simulink model "Arm6Dof"  (R2018b)
settings: Solver=VariableStepAuto  StartTime=0.0  StopTime=inf  RelTol=1e-3
undefined symbols (not defined in the file or in its folder): asm_Arm6Dof, bottom, link1, link2, link3, link4, link5, linke, RootGround, RootPart
libraries: mblibv1 x25, simulink x7
settings Model: Creator=Administrator  LastModifiedBy=Administrator
settings SimMechanicsCC: VisOnUpdateDiagram=on  VisDuringSimulation=on

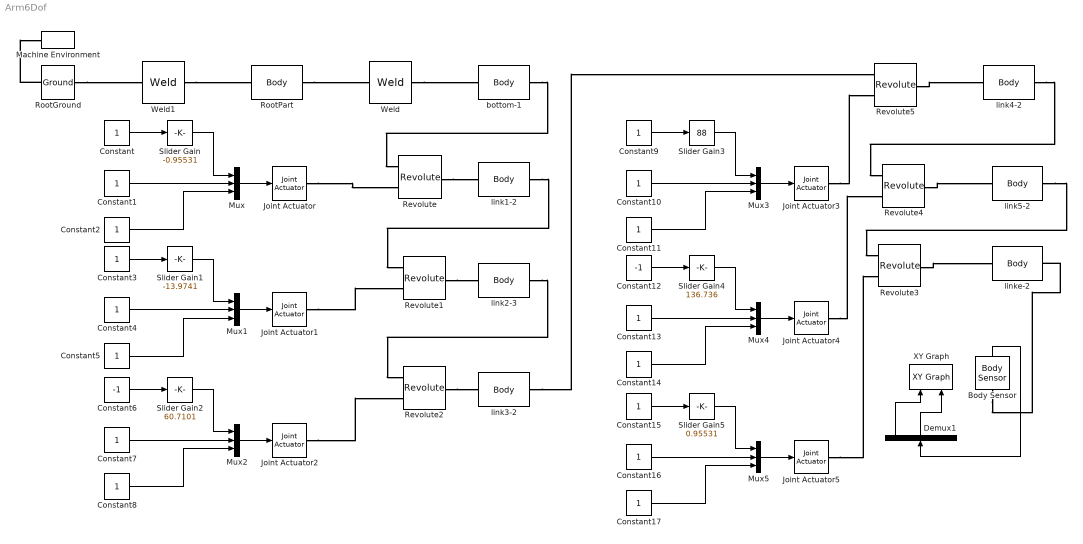
== system Arm6Dof ==
  Body Sensor : mblibv1/Sensors &  Actuators/Body Sensor  UpdateFromCAD=off  PhysicalDomain=Mechanical  PortType=blob  Muxed=on  Pose=off  Angle=on  AngleUnits=deg  ArcVelocity=off  ArcVelocityUnits=deg/s  ArcAcceleration=off  ArcAccelerationUnits=deg/s^2  CoordPosition=on  CoordPositionUnits=mm  Velocity=off  VelocityUnits=m/s  Acceleration=off  AccelerationUnits=m/s^2  Quaternion=on  QuaternionDT=off  QuaternionDDT=off  QuaternionUnits=off  OutputVector=[1]  ActiveIO=on  Width=3  DialogClass=MechanicalSensorBlock  ReferenceFrame=Absolute (World)
      settings: SourceProductName=Simscape  SourceProductBaseCode=SS
  Constant{,1..5,7..11,13..17} (16 alike) : Constant
  Constant12 : Constant  Value=-1
  Constant6 : Constant  Value=-1
  Demux1 : Demux  Outputs=3
  Joint Actuator{,1..5} (6 alike) : mblibv1/Sensors &  Actuators/Joint Actuator  UpdateFromCAD=off  PhysicalDomain=Mechanical  PortType=blob  ActuationStyle=Motion  AngleUnits=deg  ArcVelocityUnits=deg/s  ArcAccelerationUnits=deg/s^2  CoordPositionUnits=m  VelocityUnits=m/s  AccelerationUnits=m/s^2  ForceUnits=N  TorqueUnits=N*m  ActiveIO=on  Width=3  DialogClass=MechanicalActuatorBlock  Primitive=R1  ReferenceFrame=Absolute (World)
      settings: SourceProductName=Simscape  SourceProductBaseCode=SS
  Machine Environment : mblibv1/Bodies/Machine Environment  PortType=env  PhysicalDomain=Mechanical  DialogTemplateClass=MECH.MachineEnvironment  SyncWhenCopied=off  Gravity=[0 -9.81 0]  GravityUnits=m/s^2  GravityAsSignal=off  Dimensionality=Auto-detect  AnalysisType=Forward dynamics  LinearAssemblyTolerance=1e-3  LinearAssemblyToleranceUnits=m  AngularAssemblyTolerance=1e-3  AngularAssemblyToleranceUnits=rad  ConstraintSolverType=Stabilizing  ConstraintRelTolerance=1e-4  ConstraintAbsTolerance=1e-4  UseRobustSingularityHandling=off  RedundancyAnalysisToleranceType=Automatically select tolerance  RedundancyAnalysisTolerance=1e-14  StatePerturbationType=Fixed  PerturbationSize=1e-5  VisualizeMachine=on  BodyVisualizationType=Use model default body geometries  BodyColorSelMode=Use model default  DefaultBodyColor=[1 0 0]
      settings: SourceProductName=Simscape  SourceProductBaseCode=SS
  Mux{,1..5} (6 alike) : Mux  Inputs=3
  Revolute : mblibv1/Joints/Revolute  LConnTagsString=__newl0|SA1  RConnTagsString=__newr0  UpdateFromCAD=on  PMImportedID=bottom-1:-:link1-2  NumSAPorts=1  CutJoint=off  MarkAsCut=off  Primitives=prismatic  PrimitiveProps=R1$World$[0,0,1]$revolute  DialogClass=JointBlock  R1Axis=[0,0,1]
      settings: SourceProductName=Simscape  SourceProductBaseCode=SS
  Revolute1 : mblibv1/Joints/Revolute  LConnTagsString=__newl0|SA1  RConnTagsString=__newr0  UpdateFromCAD=on  PMImportedID=link1-2:-:link2-3  NumSAPorts=1  CutJoint=off  MarkAsCut=off  Primitives=prismatic  PrimitiveProps=R1$World$[0,1,0]$revolute  DialogClass=JointBlock  R1Axis=[0,1,0]
      settings: SourceProductName=Simscape  SourceProductBaseCode=SS
  Revolute2 : mblibv1/Joints/Revolute  LConnTagsString=__newl0|SA1  RConnTagsString=__newr0  UpdateFromCAD=on  PMImportedID=link2-3:-:link3-2  NumSAPorts=1  CutJoint=off  MarkAsCut=off  Primitives=prismatic  PrimitiveProps=R1$World$[0,-1,0]$revolute  DialogClass=JointBlock  R1Axis=[0,-1,0]
      settings: SourceProductName=Simscape  SourceProductBaseCode=SS
  Revolute3 : mblibv1/Joints/Revolute  LConnTagsString=__newl0|SA1  RConnTagsString=__newr0  UpdateFromCAD=on  PMImportedID=link5-2:-:linke-2  NumSAPorts=1  CutJoint=off  MarkAsCut=off  Primitives=prismatic  PrimitiveProps=R1$World$[1,0,0]$revolute  DialogClass=JointBlock  R1Axis=[1,0,0]
      settings: SourceProductName=Simscape  SourceProductBaseCode=SS
  Revolute4 : mblibv1/Joints/Revolute  LConnTagsString=__newl0|SA1  RConnTagsString=__newr0  UpdateFromCAD=on  PMImportedID=link4-2:-:link5-2  NumSAPorts=1  CutJoint=off  MarkAsCut=off  Primitives=prismatic  PrimitiveProps=R1$World$[0,-1,0]$revolute  DialogClass=JointBlock  R1Axis=[0,-1,0]
      settings: SourceProductName=Simscape  SourceProductBaseCode=SS
  Revolute5 : mblibv1/Joints/Revolute  LConnTagsString=__newl0|SA1  RConnTagsString=__newr0  UpdateFromCAD=on  PMImportedID=link3-2:-:link4-2  NumSAPorts=1  CutJoint=off  MarkAsCut=off  Primitives=prismatic  PrimitiveProps=R1$World$[1,0,0]$revolute  DialogClass=JointBlock  R1Axis=[1,0,0]
      settings: SourceProductName=Simscape  SourceProductBaseCode=SS
  RootGround : mblibv1/Bodies/Ground  UpdateFromCAD=on  PMImportedID=RootGround  LeftPortType=env  RightPortType=workingframe  PhysicalDomain=Mechanical  DialogClass=GroundBlock  CoordPosition=[0.0237894,0.00138772,0.108536]  CoordPositionUnits=m  StateVectorMgrId=0  MachineId=[1 0]  ShowEnvPort=on  ParameterChecksum=[465685806, 464748915, 4149600887, 3518869036]  TopologyChecksum=[603143340, 271073404, 1386402031, 4009897821]
      settings: SourceProductName=Simscape  SourceProductBaseCode=SS
  RootPart : mblibv1/Bodies/Body  LConnTagsString=CS3  RConnTagsString=CS2  UpdateFromCAD=on  PMImportedID=asm_Arm6Dof/RootPart  DialogClass=MechanicalBodyBlock  Mass=0  MassUnits=kg  InertiaUnits=kg*m^2  Inertia=[0,0,0;0,0,0;0,0,0]  Shape=Cylinder  ShapeDims=[1 1]  ShapeUnits=m  ShapeUse=false  Density=1  DensityUnits=kg/m^3  DensityUse=false  GraphicsMode=MACHINE_DEFAULT  BodyColorSelMode=MACHINE_DEFAULT  BodyColor=[1;0;0]  AttachedToCS=CS1  CG=Right$CG$[0.0237894 0.00138772 0.108536]$WORLD$WORLD$m$[1 0 0;0 1 0;0 0 1]$3x3 Transform$rad$WORLD$false$asm_Arm6Dof/RootPart::CG(AUTOGEN)  WorkingFrames=Right$CS1$[0 0 0]$WORLD$WORLD$m$[1 0 0;0 1 0;0 0 1]$3x3 Transform$rad$WORLD$false$asm_Arm6Dof/RootPart::CS1(AUTOGEN)#Right$CS2$[0 0 0.005]$WORLD$WORLD$m$[1 0 0;0 1 0;0 0 1]$3x3 Transform$rad$WORLD$true$asm_Arm6Dof/RootPart:-:bottom-1::asm_Arm6Dof/RootPart(AUTOGEN)#Left$CS3$[0.0237894 0.00138772 0.108536]$WORLD$WORLD$m$[1 0 0;0 1 0;0 0 1]$3x3 Transform$rad$WORLD$true$RootGround:-:asm_Arm6Dof/RootPart::asm_Arm6Dof/RootPart(AUTOGEN)  CGPos=[0.0237894 0.00138772 0.108536]  CGRot=[1 0 0;0 1 0;0 0 1]  CS0Pos=[]  CS0Rot=[]  CS1Pos=[0 0 0]  CS1Rot=[1 0 0;0 1 0;0 0 1]  CS2Pos=[0 0 0.005]  CS2Rot=[1 0 0;0 1 0;0 0 1]  CS3Pos=[0.0237894 0.00138772 0.108536]  CS3Rot=[1 0 0;0 1 0;0 0 1]  CS4Pos=[]  CS4Rot=[]  CS5Pos=[]  CS5Rot=[]  CS6Pos=[]  CS6Rot=[]  CS7Pos=[]  CS7Rot=[]  CS8Pos=[]  CS8Rot=[]  CS9Pos=[]  CS9Rot=[]  CS10Pos=[]  CS10Rot=[]  CS11Pos=[]  CS11Rot=[]  CS12Pos=[]  CS12Rot=[]  CS13Pos=[]  CS13Rot=[]  CS14Pos=[]  CS14Rot=[]  CS15Pos=[]  CS15Rot=[]  CS16Pos=[]  CS16Rot=[]  CS17Pos=[]  CS17Rot=[]  CS18Pos=[]  CS18Rot=[]  CS19Pos=[]  CS19Rot=[]  CS20Pos=[]  CS20Rot=[]
      settings: SourceProductName=Simscape  SourceProductBaseCode=SS
  Slider Gain : simulink/Math Operations/Slider Gain  gain=-0.95531  low=-180  high=180
  Slider Gain1 : simulink/Math Operations/Slider Gain  gain=-13.9741  low=-180  high=180
  Slider Gain2 : simulink/Math Operations/Slider Gain  gain=60.7101  low=-180  high=180
  Slider Gain3 : simulink/Math Operations/Slider Gain  gain=88  low=-180  high=180
  Slider Gain4 : simulink/Math Operations/Slider Gain  gain=136.736  low=-180  high=180
  Slider Gain5 : simulink/Math Operations/Slider Gain  gain=0.95531  low=-180  high=180
  Weld : mblibv1/Joints/Weld  LConnTagsString=__newl0  RConnTagsString=__newr0  UpdateFromCAD=on  PMImportedID=asm_Arm6Dof/RootPart:-:bottom-1  NumSAPorts=0  CutJoint=off  MarkAsCut=off  Primitives=weld  PrimitiveProps=W$WORLD$[0.57735,0.57735,0.57735]$weld  DialogClass=JointBlock  WAxis=[0.57735,0.57735,0.57735]
      settings: SourceProductName=Simscape  SourceProductBaseCode=SS
  Weld1 : mblibv1/Joints/Weld  LConnTagsString=__newl0  RConnTagsString=__newr0  UpdateFromCAD=on  PMImportedID=RootGround:-:asm_Arm6Dof/RootPart  NumSAPorts=0  CutJoint=off  MarkAsCut=off  Primitives=weld  PrimitiveProps=W$WORLD$[0.57735,0.57735,0.57735]$weld  DialogClass=JointBlock  WAxis=[0.57735,0.57735,0.57735]
      settings: SourceProductName=Simscape  SourceProductBaseCode=SS
  XY Graph : simulink/Sinks/XY Graph  xmin=-300  xmax=300  ymin=-300  ymax=300  st=1
  bottom-1 : mblibv1/Bodies/Body  LConnTagsString=CS2  RConnTagsString=CS3  UpdateFromCAD=on  PMImportedID=bottom-1  DialogClass=MechanicalBodyBlock  Mass=0.0989551  MassUnits=kg  InertiaUnits=kg*m^2  Inertia=[8.41493e-05,0,0;0,8.41493e-05,0;0,0,0.000166649]  Shape=Cylinder  ShapeDims=[1 1]  ShapeUnits=m  ShapeUse=false  Density=1  DensityUnits=kg/m^3  DensityUse=false  GraphicsMode=GFXFILE  GraphicsFileName=asm_Arm6Dof - bottom-1.STL  BodyColorSelMode=COLORPALETTE  BodyColor=[0.752941;0.752941;0.752941]  AttachedToCS=CS1  CG=Right$CG$[0 0 0.005]$WORLD$WORLD$m$[1 0 0;0 1 0;0 0 1]$3x3 Transform$rad$WORLD$false$bottom-1::CG(AUTOGEN)  WorkingFrames=Right$CS1$[0 0 0]$WORLD$WORLD$m$[1 0 0;0 1 0;0 0 1]$3x3 Transform$rad$WORLD$false$bottom-1::CS1(AUTOGEN)#Left$CS2$[0 0 0.005]$WORLD$WORLD$m$[1 0 0;0 1 0;0 0 1]$3x3 Transform$rad$WORLD$true$asm_Arm6Dof/RootPart:-:bottom-1::bottom-1(AUTOGEN)#Right$CS3$[0 0 0.01]$WORLD$WORLD$m$[1 0 0;0 1 0;0 0 1]$3x3 Transform$rad$WORLD$true$bottom-1:-:link1-2::bottom-1(AUTOGEN)  CGPos=[0 0 0.005]  CGRot=[1 0 0;0 1 0;0 0 1]  CS0Pos=[]  CS0Rot=[]  CS1Pos=[0 0 0]  CS1Rot=[1 0 0;0 1 0;0 0 1]  CS2Pos=[0 0 0.005]  CS2Rot=[1 0 0;0 1 0;0 0 1]  CS3Pos=[0 0 0.01]  CS3Rot=[1 0 0;0 1 0;0 0 1]  CS4Pos=[]  CS4Rot=[]  CS5Pos=[]  CS5Rot=[]  CS6Pos=[]  CS6Rot=[]  CS7Pos=[]  CS7Rot=[]  CS8Pos=[]  CS8Rot=[]  CS9Pos=[]  CS9Rot=[]  CS10Pos=[]  CS10Rot=[]  CS11Pos=[]  CS11Rot=[]  CS12Pos=[]  CS12Rot=[]  CS13Pos=[]  CS13Rot=[]  CS14Pos=[]  CS14Rot=[]  CS15Pos=[]  CS15Rot=[]  CS16Pos=[]  CS16Rot=[]  CS17Pos=[]  CS17Rot=[]  CS18Pos=[]  CS18Rot=[]  CS19Pos=[]  CS19Rot=[]  CS20Pos=[]  CS20Rot=[]
      settings: SourceProductName=Simscape  SourceProductBaseCode=SS
  link1-2 : mblibv1/Bodies/Body  LConnTagsString=CS2  RConnTagsString=CS3  UpdateFromCAD=on  PMImportedID=link1-2  DialogClass=MechanicalBodyBlock  Mass=0.27764  MassUnits=kg  InertiaUnits=kg*m^2  Inertia=[0.000579936,9.11984e-05,0;9.11984e-05,0.000159357,0;0,0,0.000651379]  Shape=Cylinder  ShapeDims=[1 1]  ShapeUnits=m  ShapeUse=false  Density=1  DensityUnits=kg/m^3  DensityUse=false  GraphicsMode=GFXFILE  GraphicsFileName=asm_Arm6Dof - link1-2.STL  BodyColorSelMode=COLORPALETTE  BodyColor=[1;0.152941;0.027451]  AttachedToCS=CS1  CG=Right$CG$[0.00665144 0 0.0836156]$WORLD$WORLD$m$[1 0 0;0 0 1;0 -1 0]$3x3 Transform$rad$WORLD$false$link1-2::CG(AUTOGEN)  WorkingFrames=Right$CS1$[0.047 0 0.133]$WORLD$WORLD$m$[1 0 0;0 0 1;0 -1 0]$3x3 Transform$rad$WORLD$false$link1-2::CS1(AUTOGEN)#Left$CS2$[0 0 0.01]$WORLD$WORLD$m$[1 0 0;0 1 0;0 0 1]$3x3 Transform$rad$WORLD$true$bottom-1:-:link1-2::link1-2(AUTOGEN)#Right$CS3$[0.047 -0.0055 0.133]$WORLD$WORLD$m$[1 0 0;0 1 0;0 0 1]$3x3 Transform$rad$WORLD$true$link1-2:-:link2-3::link1-2(AUTOGEN)  CGPos=[0.00665144 0 0.0836156]  CGRot=[1 0 0;0 0 1;0 -1 0]  CS0Pos=[]  CS0Rot=[]  CS1Pos=[0.047 0 0.133]  CS1Rot=[1 0 0;0 0 1;0 -1 0]  CS2Pos=[0 0 0.01]  CS2Rot=[1 0 0;0 1 0;0 0 1]  CS3Pos=[0.047 -0.0055 0.133]  CS3Rot=[1 0 0;0 1 0;0 0 1]  CS4Pos=[]  CS4Rot=[]  CS5Pos=[]  CS5Rot=[]  CS6Pos=[]  CS6Rot=[]  CS7Pos=[]  CS7Rot=[]  CS8Pos=[]  CS8Rot=[]  CS9Pos=[]  CS9Rot=[]  CS10Pos=[]  CS10Rot=[]  CS11Pos=[]  CS11Rot=[]  CS12Pos=[]  CS12Rot=[]  CS13Pos=[]  CS13Rot=[]  CS14Pos=[]  CS14Rot=[]  CS15Pos=[]  CS15Rot=[]  CS16Pos=[]  CS16Rot=[]  CS17Pos=[]  CS17Rot=[]  CS18Pos=[]  CS18Rot=[]  CS19Pos=[]  CS19Rot=[]  CS20Pos=[]  CS20Rot=[]
      settings: SourceProductName=Simscape  SourceProductBaseCode=SS
  link2-3 : mblibv1/Bodies/Body  LConnTagsString=CS2  RConnTagsString=CS3  UpdateFromCAD=on  PMImportedID=link2-3  DialogClass=MechanicalBodyBlock  Mass=0.0336821  MassUnits=kg  InertiaUnits=kg*m^2  Inertia=[2.11186e-06,0,0;0,4.45663e-05,0;0,0,4.59989e-05]  Shape=Cylinder  ShapeDims=[1 1]  ShapeUnits=m  ShapeUse=false  Density=1  DensityUnits=kg/m^3  DensityUse=false  GraphicsMode=GFXFILE  GraphicsFileName=asm_Arm6Dof - link2-3.STL  BodyColorSelMode=COLORPALETTE  BodyColor=[0.592157;1;0.898039]  AttachedToCS=CS1  CG=Right$CG$[0.047 0 0.187609]$WORLD$WORLD$m$[0 1 0;0 0 1;1 0 0]$3x3 Transform$rad$WORLD$false$link2-3::CG(AUTOGEN)  WorkingFrames=Right$CS1$[0.047 0 0.242832]$WORLD$WORLD$m$[0 1 0;0 0 1;1 0 0]$3x3 Transform$rad$WORLD$false$link2-3::CS1(AUTOGEN)#Left$CS2$[0.047 -0.0055 0.133]$WORLD$WORLD$m$[1 0 0;0 1 0;0 0 1]$3x3 Transform$rad$WORLD$true$link1-2:-:link2-3::link2-3(AUTOGEN)#Right$CS3$[0.047 -0.0055 0.243]$WORLD$WORLD$m$[1 0 0;0 1 0;0 0 1]$3x3 Transform$rad$WORLD$true$link2-3:-:link3-2::link2-3(AUTOGEN)  CGPos=[0.047 0 0.187609]  CGRot=[0 1 0;0 0 1;1 0 0]  CS0Pos=[]  CS0Rot=[]  CS1Pos=[0.047 0 0.242832]  CS1Rot=[0 1 0;0 0 1;1 0 0]  CS2Pos=[0.047 -0.0055 0.133]  CS2Rot=[1 0 0;0 1 0;0 0 1]  CS3Pos=[0.047 -0.0055 0.243]  CS3Rot=[1 0 0;0 1 0;0 0 1]  CS4Pos=[]  CS4Rot=[]  CS5Pos=[]  CS5Rot=[]  CS6Pos=[]  CS6Rot=[]  CS7Pos=[]  CS7Rot=[]  CS8Pos=[]  CS8Rot=[]  CS9Pos=[]  CS9Rot=[]  CS10Pos=[]  CS10Rot=[]  CS11Pos=[]  CS11Rot=[]  CS12Pos=[]  CS12Rot=[]  CS13Pos=[]  CS13Rot=[]  CS14Pos=[]  CS14Rot=[]  CS15Pos=[]  CS15Rot=[]  CS16Pos=[]  CS16Rot=[]  CS17Pos=[]  CS17Rot=[]  CS18Pos=[]  CS18Rot=[]  CS19Pos=[]  CS19Rot=[]  CS20Pos=[]  CS20Rot=[]
      settings: SourceProductName=Simscape  SourceProductBaseCode=SS
  link3-2 : mblibv1/Bodies/Body  LConnTagsString=CS2  RConnTagsString=CS3  UpdateFromCAD=on  PMImportedID=link3-2  DialogClass=MechanicalBodyBlock  Mass=0.0391453  MassUnits=kg  InertiaUnits=kg*m^2  Inertia=[1.23557e-05,-1.48864e-07,2.38665e-06;-1.48864e-07,1.50069e-05,3.39114e-08;2.38665e-06,3.39114e-08,2.14222e-05]  Shape=Cylinder  ShapeDims=[1 1]  ShapeUnits=m  ShapeUse=false  Density=1  DensityUnits=kg/m^3  DensityUse=false  GraphicsMode=GFXFILE  GraphicsFileName=asm_Arm6Dof - link3-2.STL  BodyColorSelMode=COLORPALETTE  BodyColor=[1;1;0]  AttachedToCS=CS1  CG=Right$CG$[0.0419685 0.00763392 0.258957]$WORLD$WORLD$m$[0 0 1;0 -1 0;1 0 0]$3x3 Transform$rad$WORLD$false$link3-2::CG(AUTOGEN)  WorkingFrames=Right$CS1$[0.047 0.00743997 0.269]$WORLD$WORLD$m$[0 0 1;0 -1 0;1 0 0]$3x3 Transform$rad$WORLD$false$link3-2::CS1(AUTOGEN)#Left$CS2$[0.047 -0.0055 0.243]$WORLD$WORLD$m$[1 0 0;0 1 0;0 0 1]$3x3 Transform$rad$WORLD$true$link2-3:-:link3-2::link3-2(AUTOGEN)#Right$CS3$[0.047 0.00743997 0.269]$WORLD$WORLD$m$[1 0 0;0 1 0;0 0 1]$3x3 Transform$rad$WORLD$true$link3-2:-:link4-2::link3-2(AUTOGEN)  CGPos=[0.0419685 0.00763392 0.258957]  CGRot=[0 0 1;0 -1 0;1 0 0]  CS0Pos=[]  CS0Rot=[]  CS1Pos=[0.047 0.00743997 0.269]  CS1Rot=[0 0 1;0 -1 0;1 0 0]  CS2Pos=[0.047 -0.0055 0.243]  CS2Rot=[1 0 0;0 1 0;0 0 1]  CS3Pos=[0.047 0.00743997 0.269]  CS3Rot=[1 0 0;0 1 0;0 0 1]  CS4Pos=[]  CS4Rot=[]  CS5Pos=[]  CS5Rot=[]  CS6Pos=[]  CS6Rot=[]  CS7Pos=[]  CS7Rot=[]  CS8Pos=[]  CS8Rot=[]  CS9Pos=[]  CS9Rot=[]  CS10Pos=[]  CS10Rot=[]  CS11Pos=[]  CS11Rot=[]  CS12Pos=[]  CS12Rot=[]  CS13Pos=[]  CS13Rot=[]  CS14Pos=[]  CS14Rot=[]  CS15Pos=[]  CS15Rot=[]  CS16Pos=[]  CS16Rot=[]  CS17Pos=[]  CS17Rot=[]  CS18Pos=[]  CS18Rot=[]  CS19Pos=[]  CS19Rot=[]  CS20Pos=[]  CS20Rot=[]
      settings: SourceProductName=Simscape  SourceProductBaseCode=SS
  link4-2 : mblibv1/Bodies/Body  LConnTagsString=CS3  RConnTagsString=CS2  UpdateFromCAD=on  PMImportedID=link4-2  DialogClass=MechanicalBodyBlock  Mass=0.0400295  MassUnits=kg  InertiaUnits=kg*m^2  Inertia=[5.11182e-05,0,0;0,6.5069e-06,0;0,0,4.61139e-05]  Shape=Cylinder  ShapeDims=[1 1]  ShapeUnits=m  ShapeUse=false  Density=1  DensityUnits=kg/m^3  DensityUse=false  GraphicsMode=GFXFILE  GraphicsFileName=asm_Arm6Dof - link4-2.STL  BodyColorSelMode=COLORPALETTE  BodyColor=[0;0.501961;1]  AttachedToCS=CS1  CG=Right$CG$[0.116646 0.00743997 0.269]$WORLD$WORLD$m$[0 1 0;0 0 1;1 0 0]$3x3 Transform$rad$WORLD$false$link4-2::CG(AUTOGEN)  WorkingFrames=Right$CS1$[0.1645 0.00743997 0.269]$WORLD$WORLD$m$[0 1 0;0 0 1;1 0 0]$3x3 Transform$rad$WORLD$false$link4-2::CS1(AUTOGEN)#Right$CS2$[0.1645 -0.01756 0.269]$WORLD$WORLD$m$[1 0 0;0 1 0;0 0 1]$3x3 Transform$rad$WORLD$true$link4-2:-:link5-2::link4-2(AUTOGEN)#Left$CS3$[0.047 0.00743997 0.269]$WORLD$WORLD$m$[1 0 0;0 1 0;0 0 1]$3x3 Transform$rad$WORLD$true$link3-2:-:link4-2::link4-2(AUTOGEN)  CGPos=[0.116646 0.00743997 0.269]  CGRot=[0 1 0;0 0 1;1 0 0]  CS0Pos=[]  CS0Rot=[]  CS1Pos=[0.1645 0.00743997 0.269]  CS1Rot=[0 1 0;0 0 1;1 0 0]  CS2Pos=[0.1645 -0.01756 0.269]  CS2Rot=[1 0 0;0 1 0;0 0 1]  CS3Pos=[0.047 0.00743997 0.269]  CS3Rot=[1 0 0;0 1 0;0 0 1]  CS4Pos=[]  CS4Rot=[]  CS5Pos=[]  CS5Rot=[]  CS6Pos=[]  CS6Rot=[]  CS7Pos=[]  CS7Rot=[]  CS8Pos=[]  CS8Rot=[]  CS9Pos=[]  CS9Rot=[]  CS10Pos=[]  CS10Rot=[]  CS11Pos=[]  CS11Rot=[]  CS12Pos=[]  CS12Rot=[]  CS13Pos=[]  CS13Rot=[]  CS14Pos=[]  CS14Rot=[]  CS15Pos=[]  CS15Rot=[]  CS16Pos=[]  CS16Rot=[]  CS17Pos=[]  CS17Rot=[]  CS18Pos=[]  CS18Rot=[]  CS19Pos=[]  CS19Rot=[]  CS20Pos=[]  CS20Rot=[]
      settings: SourceProductName=Simscape  SourceProductBaseCode=SS
  link5-2 : mblibv1/Bodies/Body  LConnTagsString=CS3  RConnTagsString=CS2  UpdateFromCAD=on  PMImportedID=link5-2  DialogClass=MechanicalBodyBlock  Mass=0.0128471  MassUnits=kg  InertiaUnits=kg*m^2  Inertia=[1.62612e-06,0,0;0,1.33365e-06,0;0,0,1.78245e-06]  Shape=Cylinder  ShapeDims=[1 1]  ShapeUnits=m  ShapeUse=false  Density=1  DensityUnits=kg/m^3  DensityUse=false  GraphicsMode=GFXFILE  GraphicsFileName=asm_Arm6Dof - link5-2.STL  BodyColorSelMode=COLORPALETTE  BodyColor=[1;0.501961;1]  AttachedToCS=CS1  CG=Right$CG$[0.162574 0.00743997 0.269]$WORLD$WORLD$m$[0 0 1;0 -1 0;1 0 0]$3x3 Transform$rad$WORLD$false$link5-2::CG(AUTOGEN)  WorkingFrames=Right$CS1$[0.1645 0.00743997 0.269]$WORLD$WORLD$m$[0 0 1;0 -1 0;1 0 0]$3x3 Transform$rad$WORLD$false$link5-2::CS1(AUTOGEN)#Right$CS2$[0.1645 0.00743997 0.269]$WORLD$WORLD$m$[1 0 0;0 1 0;0 0 1]$3x3 Transform$rad$WORLD$true$link5-2:-:linke-2::link5-2(AUTOGEN)#Left$CS3$[0.1645 -0.01756 0.269]$WORLD$WORLD$m$[1 0 0;0 1 0;0 0 1]$3x3 Transform$rad$WORLD$true$link4-2:-:link5-2::link5-2(AUTOGEN)  CGPos=[0.162574 0.00743997 0.269]  CGRot=[0 0 1;0 -1 0;1 0 0]  CS0Pos=[]  CS0Rot=[]  CS1Pos=[0.1645 0.00743997 0.269]  CS1Rot=[0 0 1;0 -1 0;1 0 0]  CS2Pos=[0.1645 0.00743997 0.269]  CS2Rot=[1 0 0;0 1 0;0 0 1]  CS3Pos=[0.1645 -0.01756 0.269]  CS3Rot=[1 0 0;0 1 0;0 0 1]  CS4Pos=[]  CS4Rot=[]  CS5Pos=[]  CS5Rot=[]  CS6Pos=[]  CS6Rot=[]  CS7Pos=[]  CS7Rot=[]  CS8Pos=[]  CS8Rot=[]  CS9Pos=[]  CS9Rot=[]  CS10Pos=[]  CS10Rot=[]  CS11Pos=[]  CS11Rot=[]  CS12Pos=[]  CS12Rot=[]  CS13Pos=[]  CS13Rot=[]  CS14Pos=[]  CS14Rot=[]  CS15Pos=[]  CS15Rot=[]  CS16Pos=[]  CS16Rot=[]  CS17Pos=[]  CS17Rot=[]  CS18Pos=[]  CS18Rot=[]  CS19Pos=[]  CS19Rot=[]  CS20Pos=[]  CS20Rot=[]
      settings: SourceProductName=Simscape  SourceProductBaseCode=SS
  linke-2 : mblibv1/Bodies/Body  LConnTagsString=CS2  RConnTagsString=CS1  UpdateFromCAD=on  PMImportedID=linke-2  DialogClass=MechanicalBodyBlock  Mass=0.000797457  MassUnits=kg  InertiaUnits=kg*m^2  Inertia=[3.72849e-08,0,0;0,3.72648e-08,-1.51123e-10;0,-1.51123e-10,5.72875e-09]  Shape=Cylinder  ShapeDims=[1 1]  ShapeUnits=m  ShapeUse=false  Density=1  DensityUnits=kg/m^3  DensityUse=false  GraphicsMode=GFXFILE  GraphicsFileName=asm_Arm6Dof - linke-2.STL  BodyColorSelMode=COLORPALETTE  BodyColor=[0 1 0]  AttachedToCS=CS1  CG=Right$CG$[0.172855 0.00742883 0.269]$WORLD$WORLD$m$[0 0 1;0 -1 0;1 0 0]$3x3 Transform$rad$WORLD$false$linke-2::CG(AUTOGEN)  WorkingFrames=Right$CS1$[0.1925 0.00743997 0.269]$WORLD$WORLD$m$[0 0 1;0 -1 0;1 0 0]$3x3 Transform$rad$WORLD$true$linke-2::CS1(AUTOGEN)#Left$CS2$[0.1645 0.00743997 0.269]$WORLD$WORLD$m$[1 0 0;0 1 0;0 0 1]$3x3 Transform$rad$WORLD$true$link5-2:-:linke-2::linke-2(AUTOGEN)  CGPos=[0.172855 0.00742883 0.269]  CGRot=[0 0 1;0 -1 0;1 0 0]  CS0Pos=[]  CS0Rot=[]  CS1Pos=[0.1925 0.00743997 0.269]  CS1Rot=[0 0 1;0 -1 0;1 0 0]  CS2Pos=[0.1645 0.00743997 0.269]  CS2Rot=[1 0 0;0 1 0;0 0 1]  CS3Pos=[]  CS3Rot=[]  CS4Pos=[]  CS4Rot=[]  CS5Pos=[]  CS5Rot=[]  CS6Pos=[]  CS6Rot=[]  CS7Pos=[]  CS7Rot=[]  CS8Pos=[]  CS8Rot=[]  CS9Pos=[]  CS9Rot=[]  CS10Pos=[]  CS10Rot=[]  CS11Pos=[]  CS11Rot=[]  CS12Pos=[]  CS12Rot=[]  CS13Pos=[]  CS13Rot=[]  CS14Pos=[]  CS14Rot=[]  CS15Pos=[]  CS15Rot=[]  CS16Pos=[]  CS16Rot=[]  CS17Pos=[]  CS17Rot=[]  CS18Pos=[]  CS18Rot=[]  CS19Pos=[]  CS19Rot=[]  CS20Pos=[]  CS20Rot=[]
      settings: SourceProductName=Simscape  SourceProductBaseCode=SS
  wires:
  Constant5/1 -> Mux1/3
  Constant7/1 -> Mux2/2
  Constant/1 -> Slider Gain/1
  Constant6/1 -> Slider Gain2/1
  Mux1/1 -> Joint Actuator1/1
  Constant3/1 -> Slider Gain1/1
  Mux2/1 -> Joint Actuator2/1
  Slider Gain1/1 -> Mux1/1
  Constant2/1 -> Mux/3
  Constant4/1 -> Mux1/2
  Constant8/1 -> Mux2/3
  Slider Gain/1 -> Mux/1
  Constant1/1 -> Mux/2
  Mux/1 -> Joint Actuator/1
  Slider Gain2/1 -> Mux2/1
  Constant16/1 -> Mux5/2
  Constant17/1 -> Mux5/3
  Slider Gain4/1 -> Mux4/1
  Constant14/1 -> Mux4/3
  Constant9/1 -> Slider Gain3/1
  Constant11/1 -> Mux3/3
  Slider Gain5/1 -> Mux5/1
  Mux3/1 -> Joint Actuator3/1
  Constant15/1 -> Slider Gain5/1
  Constant10/1 -> Mux3/2
  Constant13/1 -> Mux4/2
  Constant12/1 -> Slider Gain4/1
  Mux4/1 -> Joint Actuator4/1
  Mux5/1 -> Joint Actuator5/1
  Slider Gain3/1 -> Mux3/1
  Demux1/2 -> XY Graph/2
  Demux1/1 -> XY Graph/1
  Body Sensor/1 -> Demux1/1
  connections:
  RootPart/RConn1 -- Weld/LConn1
  Weld/RConn1 -- bottom-1/LConn1
  bottom-1/RConn1 -- Revolute/LConn1
  Revolute/RConn1 -- link1-2/LConn1
  link1-2/RConn1 -- Revolute1/LConn1
  Revolute1/RConn1 -- link2-3/LConn1
  link2-3/RConn1 -- Revolute2/LConn1
  Revolute2/RConn1 -- link3-2/LConn1
  link5-2/RConn1 -- Revolute3/LConn1
  Revolute3/RConn1 -- linke-2/LConn1
  link4-2/RConn1 -- Revolute4/LConn1
  Revolute4/RConn1 -- link5-2/LConn1
  link3-2/RConn1 -- Revolute5/LConn1
  Revolute5/RConn1 -- link4-2/LConn1
  RootGround/RConn1 -- Weld1/LConn1
  Weld1/RConn1 -- RootPart/LConn1
  RootGround/LConn1 -- Machine Environment/RConn1
  Joint Actuator/RConn1 -- Revolute/LConn2
  Joint Actuator1/RConn1 -- Revolute1/LConn2
  Joint Actuator2/RConn1 -- Revolute2/LConn2
  Joint Actuator3/RConn1 -- Revolute5/LConn2
  Joint Actuator4/RConn1 -- Revolute4/LConn2
  Joint Actuator5/RConn1 -- Revolute3/LConn2
  Body Sensor/LConn1 -- linke-2/RConn1
